simulink model "PMSM_Sinusoidal"  (R2023a)
settings: Solver=VariableStepAuto  StartTime=0.0  StopTime=5e-3  MaxStep=5e-8  RelTol=1e-5
libraries: SLNS x4, simulink_extras x3
settings Model: Creator=Szalay  LastModifiedBy=Szalay
settings SolverCC: AlgebraicLoopSolver=TrustRegion
settings DebuggingCC: UnconnectedInputMsg=warning  UnconnectedOutputMsg=warning  UnconnectedLineMsg=warning
settings ModelReferenceCC: EnableRefExpFcnMdlSchedulingChecks=on
settings RTWCC: DLArmComputeVersion=19.05

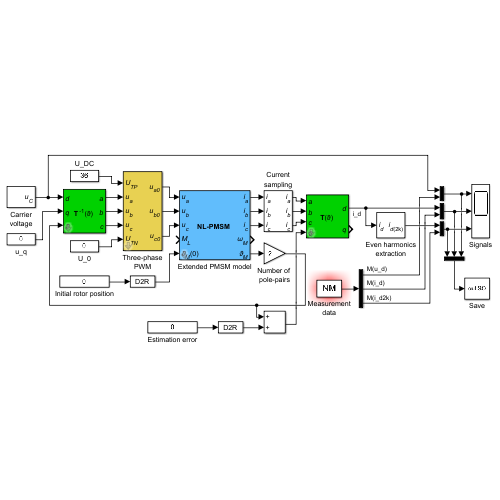
[thumbnail: Simulink's stored preview of the top-level diagram]
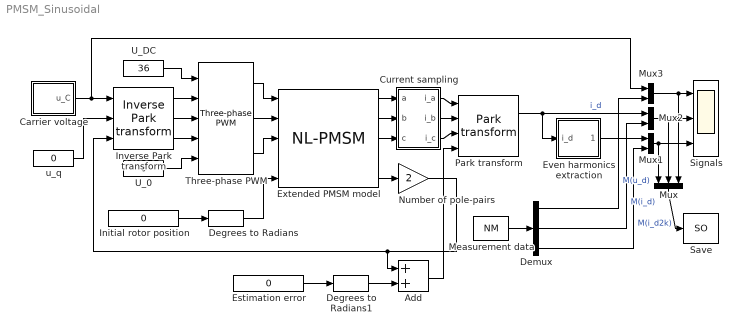
== system PMSM_Sinusoidal ==
  Add : Sum
  Carrier voltage : Subsystem
      mask Display: port_label('output', 1, '\itu_C', 'texmode', 'on');
  Current sampling : Subsystem
      mask Display:
      | port_label('input', 1, '\iti_a', 'texmode', 'on');
      | port_label('input', 2, '\iti_b', 'texmode', 'on');
      | port_label('input', 3, '\iti_c', 'texmode', 'on');
      | 
      | port_label('output', 1, '\iti_a', 'texmode', 'on');
      | port_label('output', 2, '\iti_b', 'texmode', 'on');
      | port_label('output', 3, '\iti_c', 'texmode', 'on');
  Degrees to Radians : simulink_extras/Transformations/Degrees to Radians
  Degrees to Radians1 : simulink_extras/Transformations/Degrees to Radians
  Demux : Demux  Outputs=3
  Estimation error : Constant  Value=0
  Even harmonics extraction : Subsystem
      mask Display:
      | port_label('input', 1, '\iti_d', 'texmode', 'on');
      | 
      | port_label('output', 1, '{\iti}_{{\itd} (2k)}', 'texmode', 'on');
  Extended PMSM model : SLNS/Electric machines/NL-PMSM  varZp=2  varRs=0.55  varF_PM=24.83  varLd=158  varLq=182  varG_0=0.125  varB=6.329e-3  varJ=200  i_d0=0  i_q0=0
  Initial rotor position : Constant  Value=0
  Inverse Park transform : SLNS/Transformations/Inverse Park transform  cbZero=off
  Measurement data : FromWorkspace  VariableName=NM  SampleTime=1/240000  Interpolate=off  OutputAfterFinalValue=Cyclic repetition
  Mux : Mux  Inputs=3
  Mux1 : Mux  Inputs=2
  Mux2 : Mux  Inputs=2
  Mux3 : Mux  Inputs=2
  Number of pole-pairs : Gain  Gain=2
  Park transform : SLNS/Transformations/Park transform  cbZero=off
  Save : ToWorkspace  VariableName=SO  SampleTime=1/240000
  Signals : Scope  NumInputPorts=3
  Three-phase PWM : SLNS/Power electronics/Three-phase PWM  f=40000
  U_0 : Constant  Value=0
  U_DC : Constant  Value=36
  u_q : Constant  Value=0
  wires:
  Inverse Park transform/1 -> Three-phase PWM/2
  U_0/1 -> Three-phase PWM/5
  U_DC/1 -> Three-phase PWM/1
  Inverse Park transform/2 -> Three-phase PWM/3
  Inverse Park transform/3 -> Three-phase PWM/4
  Extended PMSM model/5 -> Number of pole-pairs/1
  Initial rotor position/1 -> Degrees to Radians/1
  Degrees to Radians/1 -> Extended PMSM model/5
  Number of pole-pairs/1 -> Add/1, Inverse Park transform/3
  u_q/1 -> Inverse Park transform/2
  Three-phase PWM/1 -> Extended PMSM model/1
  Three-phase PWM/2 -> Extended PMSM model/2
  Three-phase PWM/3 -> Extended PMSM model/3
  Park transform/1 -> Mux2/1, Even harmonics extraction/1(i_d)  "i_d"
  Measurement data/1 -> Demux/1
  Demux/3 -> Mux1/2  "M(i_d2k)"
  Mux2/1 -> Mux/2, Signals/2
  Demux/2 -> Mux2/2  "M(i_d)"
  Mux1/1 -> Signals/3, Mux/1
  Demux/1 -> Mux3/2  "M(u_d)"
  Carrier voltage/1(u_C) -> Inverse Park transform/1, Mux3/1
  Mux3/1 -> Mux/3, Signals/1
  Extended PMSM model/1 -> Current sampling/1(a)
  Extended PMSM model/2 -> Current sampling/2(b)
  Extended PMSM model/3 -> Current sampling/3(c)
  Current sampling/1(i_a) -> Park transform/1
  Current sampling/2(i_b) -> Park transform/2
  Current sampling/3(i_c) -> Park transform/3
  Even harmonics extraction/1(i_d2) -> Mux1/1
  Mux/1 -> Save/1
  Estimation error/1 -> Degrees to Radians1/1
  Degrees to Radians1/1 -> Add/2
  Add/1 -> Park transform/4

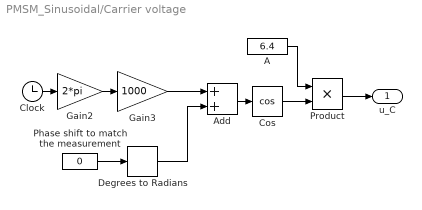
== system PMSM_Sinusoidal/Carrier voltage ==
  A : Constant  Value=6.4
  Add : Sum
  Clock : Clock
  Cos : Trigonometry  Operator=cos
  Degrees to Radians : simulink_extras/Transformations/Degrees to Radians
  Gain2 : Gain  Gain=2*pi
  Gain3 : Gain  Gain=1000
  Phase shift to match the measurement : Constant  Value=0
  Product : Product
  u_C : Outport
  wires:
  Clock/1 -> Gain2/1
  Gain2/1 -> Gain3/1
  Product/1 -> u_C/1
  Cos/1 -> Product/2
  Gain3/1 -> Add/1
  A/1 -> Product/1
  Add/1 -> Cos/1
  Phase shift to match the measurement/1 -> Degrees to Radians/1
  Degrees to Radians/1 -> Add/2

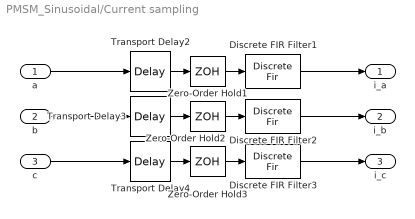
== system PMSM_Sinusoidal/Current sampling ==
  a : Inport
  b : Inport  Port=2
  c : Inport  Port=3
  Discrete FIR Filter1 : DiscreteFir  Coefficients=ones(1, 6)/6  SampleTime=1/240000
  Discrete FIR Filter2 : DiscreteFir  Coefficients=ones(1, 6)/6  SampleTime=1/240000
  Discrete FIR Filter3 : DiscreteFir  Coefficients=ones(1, 6)/6  SampleTime=1/240000
  Transport Delay2 : TransportDelay  DelayTime=1/240000/2
  Transport Delay3 : TransportDelay  DelayTime=1/240000/2
  Transport Delay4 : TransportDelay  DelayTime=1/240000/2
  Zero-Order Hold1 : ZeroOrderHold  SampleTime=1/240000
  Zero-Order Hold2 : ZeroOrderHold  SampleTime=1/240000
  Zero-Order Hold3 : ZeroOrderHold  SampleTime=1/240000
  i_a : Outport
  i_b : Outport  Port=2
  i_c : Outport  Port=3
  wires:
  Transport Delay2/1 -> Zero-Order Hold1/1
  Zero-Order Hold1/1 -> Discrete FIR Filter1/1
  Zero-Order Hold3/1 -> Discrete FIR Filter3/1
  c/1 -> Transport Delay4/1
  Zero-Order Hold2/1 -> Discrete FIR Filter2/1
  Transport Delay4/1 -> Zero-Order Hold3/1
  Transport Delay3/1 -> Zero-Order Hold2/1
  b/1 -> Transport Delay3/1
  a/1 -> Transport Delay2/1
  Discrete FIR Filter2/1 -> i_b/1
  Discrete FIR Filter1/1 -> i_a/1
  Discrete FIR Filter3/1 -> i_c/1

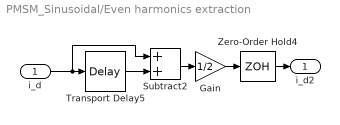
== system PMSM_Sinusoidal/Even harmonics extraction ==
  i_d : Inport
  Gain : Gain  Gain=1/2
  Subtract2 : Sum
  Transport Delay5 : TransportDelay  DelayTime=(1/240000)*240/2
  Zero-Order Hold4 : ZeroOrderHold  SampleTime=1/240000
  i_d2 : Outport
  wires:
  i_d/1 -> Subtract2/1, Transport Delay5/1
  Gain/1 -> Zero-Order Hold4/1
  Transport Delay5/1 -> Subtract2/2
  Subtract2/1 -> Gain/1
  Zero-Order Hold4/1 -> i_d2/1
